simulink model "FOCctrlBasedOnMBD"  (R2020b)
settings: Solver=FixedStepDiscrete  StartTime=0.0  StopTime=10.0  FixedStep=0.0001  RelTol=1e-3
PreLoadFcn:
  | load('structFOCMotorCrtl.mat');
InitFcn:
  | mbd_s32k_consistency_checks(bdroot(gcs));
undefined symbols (not defined in the file or in its folder): DiscIntNeverNeededParam, External, LQFP, One, Shot, TRGMUX_PDB_TRIG
libraries: mbd_s32k1xx_ec_toolbox x34, mcbcontrolslib x12, mbd_msd_ec_toolbox x1, mcbpositiondecoderlib x1
(part 2 of 2)

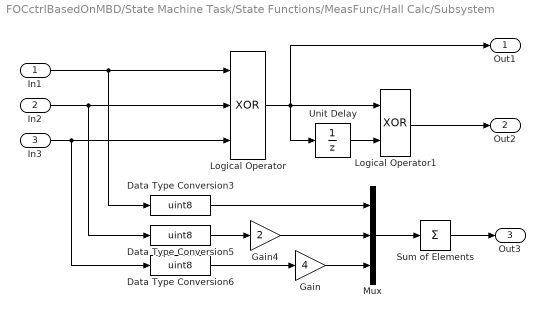
== system FOCctrlBasedOnMBD/State Machine Task/State Functions/MeasFunc/Hall Calc/Subsystem ==
  In1 : Inport
  In2 : Inport  Port=2
  In3 : Inport  Port=3
  Data Type Conversion3 : DataTypeConversion  OutDataTypeStr=uint8
  Data Type Conversion5 : DataTypeConversion  OutDataTypeStr=uint8
  Data Type Conversion6 : DataTypeConversion  OutDataTypeStr=uint8
  Gain : Gain  Gain=4  OutDataTypeStr=uint8
  Gain4 : Gain  Gain=2  OutDataTypeStr=uint8
  Logical Operator : Logic  Operator=XOR  Inputs=3  AllPortsSameDT=off  OutDataTypeStr=boolean
  Logical Operator1 : Logic  Operator=XOR  AllPortsSameDT=off  OutDataTypeStr=boolean
  Mux : Mux  Inputs=3
  Sum of Elements : Sum  Inputs=+
  Unit Delay : UnitDelay  SampleTime=-1  HasFrameUpgradeWarning=on
  Out1 : Outport
  Out2 : Outport  Port=2
  Out3 : Outport  Port=3
  wires:
  Gain4/1 -> Mux/2
  Unit Delay/1 -> Logical Operator1/2
  Logical Operator/1 -> Out1/1, Unit Delay/1, Logical Operator1/1
  In3/1 -> Data Type Conversion6/1, Logical Operator/3
  Data Type Conversion6/1 -> Gain/1
  Data Type Conversion3/1 -> Mux/1
  Gain/1 -> Mux/3
  In1/1 -> Data Type Conversion3/1, Logical Operator/1
  Mux/1 -> Sum of Elements/1
  Data Type Conversion5/1 -> Gain4/1
  In2/1 -> Data Type Conversion5/1, Logical Operator/2
  Sum of Elements/1 -> Out3/1
  Logical Operator1/1 -> Out2/1

== system FOCctrlBasedOnMBD/State Machine Task/State Functions/MeasFunc/Hall Speed Calc/If Action Subsystem ==
  note: pi/3/0.0001 = 10471.975511965977461542144610932
  Action Port : ActionPort  ActionPortLabel=if(u1 < u2)
  Constant1 : Constant  Value=10471.975511965977461542144610932  OutDataTypeStr=single
  Data Store Read1 : DataStoreRead  DataStoreName=varFOC  DataStoreElements=varFOC.Signals.Hall.HallSpd.HallEnd#varFOC.Signals.Hall.HallSpd.HallStart
  Data Store Write5 : DataStoreWrite  DataStoreName=varFOC  DataStoreElements=varFOC.Signals.Hall.HallSpd.HallSpd
  Data Type Conversion : DataTypeConversion  OutDataTypeStr=single
  Divide : Product  Inputs=*/
  Subsystem : Subsystem
  Sum : Sum  Inputs=|+-
  wires:
  Data Store Read1/1 -> Sum/1
  Data Store Read1/2 -> Sum/2
  Constant1/1 -> Divide/1
  Sum/1 -> Data Type Conversion/1
  Divide/1 -> Subsystem/1(In1)
  Subsystem/1(Out1) -> Data Store Write5/1
  Data Type Conversion/1 -> Divide/2

== system FOCctrlBasedOnMBD/State Machine Task/State Functions/MeasFunc/Hall Speed Calc/If Action Subsystem1 ==
  note: pi/3/0.0001 = 10471.975511965977461542144610932
  Action Port : ActionPort  ActionPortLabel=else
  Constant : Constant  Value=4294967295  OutDataTypeStr=uint32
  Constant1 : Constant  Value=10471.975511965977461542144610932  OutDataTypeStr=single
  Data Store Read2 : DataStoreRead  DataStoreName=varFOC  DataStoreElements=varFOC.Signals.Hall.HallSpd.HallStart#varFOC.Signals.Hall.HallSpd.HallEnd
  Data Store Write5 : DataStoreWrite  DataStoreName=varFOC  DataStoreElements=varFOC.Signals.Hall.HallSpd.HallSpd
  Data Type Conversion : DataTypeConversion  OutDataTypeStr=single
  Divide : Product  Inputs=*/
  Subsystem : Subsystem
  Sum : Sum  Inputs=|++
  Sum1 : Sum  Inputs=|+-
  wires:
  Data Store Read2/2 -> Sum/2
  Constant1/1 -> Divide/1
  Constant/1 -> Sum1/1
  Data Store Read2/1 -> Sum1/2
  Sum1/1 -> Sum/1
  Sum/1 -> Data Type Conversion/1
  Data Type Conversion/1 -> Divide/2
  Divide/1 -> Subsystem/1(In1)
  Subsystem/1(Out1) -> Data Store Write5/1

== system FOCctrlBasedOnMBD/State Machine Task/State Functions/MeasFunc/Hall Speed Calc/If Action Subsystem2 ==
  Action Port : ActionPort  ActionPortLabel=elseif(u1 == u2)
  Constant : Constant  Value=0  OutDataTypeStr=single
  Data Store Write5 : DataStoreWrite  DataStoreName=varFOC  DataStoreElements=varFOC.Signals.Hall.HallSpd.HallSpd
  wires:
  Constant/1 -> Data Store Write5/1

== system FOCctrlBasedOnMBD/State Machine Task/State Functions/NomalRunFunc/Subsystem/Subsystem ==
  In1 : Inport
  In2 : Inport  Port=2
  Constant : Constant  Value=0  OutDataTypeStr=single
  Constant1 : Constant  Value=3.1415926535897932384626433832795  OutDataTypeStr=single
  Data Store Read1 : DataStoreRead  DataStoreName=varFOC  DataStoreElements=varFOC.Signals.Current.iAlBe.iAlpha#varFOC.Signals.Current.iAlBe.iBeta
  Data Store Write2 : DataStoreWrite  DataStoreName=varFOC  DataStoreElements=varFOC.Signals.SMO.Angle#varFOC.Signals.SMO.Velocity
  Gain : Gain  Gain=12  OutDataTypeStr=single
  Gain1 : Gain  Gain=2  OutDataTypeStr=single
  Gain4 : Gain  Gain=12  OutDataTypeStr=single
  IIR Filter : mcbcontrolslib/IIR Filter  Filter_constant=0.001
      settings: SourceProductBaseCode=MT
  Sliding Mode Observer : mcbpositiondecoderlib/Sliding Mode Observer  CurrentObserverGain=1  SlidingLimit=0.01  PositionUnit=Radians  PositionDataType=single  SpeedUnit=Radians/sec  PerUnitSpeed=6000  SpeedDataType=single  BlkSampleTime=0.0001  StatorResistance=0.56  StatorInductance=4e-4  MaxApplicationSpeed=5000  PolePairs=2  MaxStatorVoltage=12  MaxStatorCurrent=2.3
      settings: SourceProductBaseCode=MT
  Sum : Sum  Inputs=-+|
  wires:
  Sliding Mode Observer/2 -> Gain1/1
  Constant1/1 -> Sum/1
  Gain4/1 -> Sliding Mode Observer/2
  Gain/1 -> Sliding Mode Observer/1
  Constant/1 -> Sliding Mode Observer/5
  Data Store Read1/1 -> Sliding Mode Observer/3
  Sum/1 -> Data Store Write2/1
  Sliding Mode Observer/1 -> Sum/2
  Data Store Read1/2 -> Sliding Mode Observer/4
  In1/1 -> Gain/1
  In2/1 -> Gain4/1
  IIR Filter/1 -> Data Store Write2/2
  Gain1/1 -> IIR Filter/1

== system FOCctrlBasedOnMBD/State Machine Task/State Functions/NomalRunFunc/Subsystem1/Subsystem ==
  Data Store Read : DataStoreRead  DataStoreName=varFOC  DataStoreElements=varFOC.MotorCtrl.CntrlReq.idReq#varFOC.Signals.Current.iDQ.iD#varFOC.Regulator.idPI.Kp#varFOC.Regulator.idPI.Ki#varFOC.Regulator.idPI.Ts
  Product : Product
  Sum : Sum  Inputs=|+-
  Out1 : Outport  OutDataTypeStr=single
  Out2 : Outport  Port=2  OutDataTypeStr=single
  Out3 : Outport  Port=3  OutDataTypeStr=single
  wires:
  Data Store Read/5 -> Product/2
  Data Store Read/1 -> Sum/1
  Data Store Read/2 -> Sum/2
  Data Store Read/3 -> Out2/1
  Data Store Read/4 -> Product/1
  Sum/1 -> Out1/1
  Product/1 -> Out3/1

== system FOCctrlBasedOnMBD/State Machine Task/State Functions/NomalRunFunc/Subsystem1/Subsystem1 ==
  Data Store Read1 : DataStoreRead  DataStoreName=varFOC  DataStoreElements=varFOC.MotorCtrl.CntrlReq.iqReq#varFOC.Signals.Current.iDQ.iQ#varFOC.Regulator.iqPI.Kp#varFOC.Regulator.iqPI.Ki#varFOC.Regulator.iqPI.Ts
  Product1 : Product
  Sum1 : Sum  Inputs=|+-
  Out1 : Outport  OutDataTypeStr=single
  Out2 : Outport  Port=2  OutDataTypeStr=single
  Out3 : Outport  Port=3  OutDataTypeStr=single
  wires:
  Sum1/1 -> Out1/1
  Data Store Read1/2 -> Sum1/2
  Data Store Read1/5 -> Product1/2
  Data Store Read1/3 -> Out2/1
  Data Store Read1/4 -> Product1/1
  Data Store Read1/1 -> Sum1/1
  Product1/1 -> Out3/1

== system FOCctrlBasedOnMBD/State Machine Task/State Functions/MeasFunc/Hall Speed Calc/If Action Subsystem/Subsystem ==
  In1 : Inport
  Constant1 : Constant  OutDataTypeStr=single
  Constant2 : Constant  Value=0.0001  OutDataTypeStr=single
  Data Store Read3 : DataStoreRead  DataStoreName=varFOC  DataStoreElements=varFOC.Signals.Hall.HallSpd.HallSpd
  Product1 : Product
  Product2 : Product
  Sum1 : Sum  Inputs=|+-
  Sum2 : Sum  Inputs=|++
  Out1 : Outport
  wires:
  Sum1/1 -> Product1/2
  Constant2/1 -> Sum1/2, Product2/1
  Constant1/1 -> Sum1/1
  Product1/1 -> Sum2/1
  Data Store Read3/1 -> Product1/1
  Sum2/1 -> Out1/1
  Product2/1 -> Sum2/2
  In1/1 -> Product2/2

== system FOCctrlBasedOnMBD/State Machine Task/State Functions/MeasFunc/Hall Speed Calc/If Action Subsystem1/Subsystem ==
  In1 : Inport
  Constant1 : Constant  OutDataTypeStr=single
  Constant2 : Constant  Value=0.0001  OutDataTypeStr=single
  Data Store Read3 : DataStoreRead  DataStoreName=varFOC  DataStoreElements=varFOC.Signals.Hall.HallSpd.HallSpd
  Product1 : Product
  Product2 : Product
  Sum1 : Sum  Inputs=|+-
  Sum2 : Sum  Inputs=|++
  Out1 : Outport
  wires:
  Sum1/1 -> Product1/2
  Constant2/1 -> Sum1/2, Product2/1
  Constant1/1 -> Sum1/1
  Product1/1 -> Sum2/1
  Data Store Read3/1 -> Product1/1
  Sum2/1 -> Out1/1
  Product2/1 -> Sum2/2
  In1/1 -> Product2/2

== stateflow chart FOCctrlBasedOnMBD/State Machine Task/Chart ==
  state ReadADC [parallel]
    ReadADCFunc;
    settings: executionOrder=1
  state StateMachine [parallel]
    settings: executionOrder=2
    state Initial
      en:
      InitFunc;
      InitDone = true;
      bind:InitFunc;
    state Ready
      en:ReadyFunc;
      du:ReadyFunc;
      bind:ReadyFunc;
    state Run
      MeasFunc;
      state Calibration
        en:CalCnt = 0;
        du:CalCnt = CalCnt + 1;CalFunc;
        bind:CalFunc;
      state NormalRun
        en:NormalRunFunc;
        du:NormalRunFunc;
        bind:NormalRunFunc;
      (default) -> Calibration
      Calibration -> NormalRun : [CalCnt > 10000]{CalCnt = 0;}
    state Faults
      en:FaultFunc;
      du:FaultFunc;
      bind:FaultFunc;
    Run -> Initial [order 1] : [~MotorOnOff]{InitDone = false;}
    (default) -> Initial : {InitDone = false;}
    Initial -> Ready [order 1] : [InitDone]
    Ready -> Run [order 1] : [MotorOnOff]
    Ready -> Faults [order 2] : [FaultSetClear]
    Faults -> Initial : [~FaultSetClear]
    Initial -> Faults [order 2] : [FaultSetClear]
    Run -> Faults [order 2] : [FaultSetClear]
  state UpdateFTM [parallel]
    UpdateFTMFunc;
    settings: executionOrder=3
  data: CalCnt local; InitDone local boolean; MotorOnOff input boolean; FaultSetClear input boolean
  events: MeasFunc output FUNCTION_CALL_EVENT; InitFunc output FUNCTION_CALL_EVENT; ReadyFunc output FUNCTION_CALL_EVENT; CalFunc output FUNCTION_CALL_EVENT; NormalRunFunc output FUNCTION_CALL_EVENT; FaultFunc output FUNCTION_CALL_EVENT; ReadADCFunc output FUNCTION_CALL_EVENT; UpdateFTMFunc output FUNCTION_CALL_EVENT
